simulink model "Three0mniwheel"  (R2020a)
settings: Solver=VariableStepAuto  StartTime=0.0  StopTime=inf  RelTol=1e-3
values from neighbouring files (symbols this model uses):
  sampleTime = 0.05    [PR_TR_parameters.m]
libraries: mobileRoboticsLib x4
settings Model: Creator=ADMIN  LastModifiedBy=RAJENDRA PHUTANE

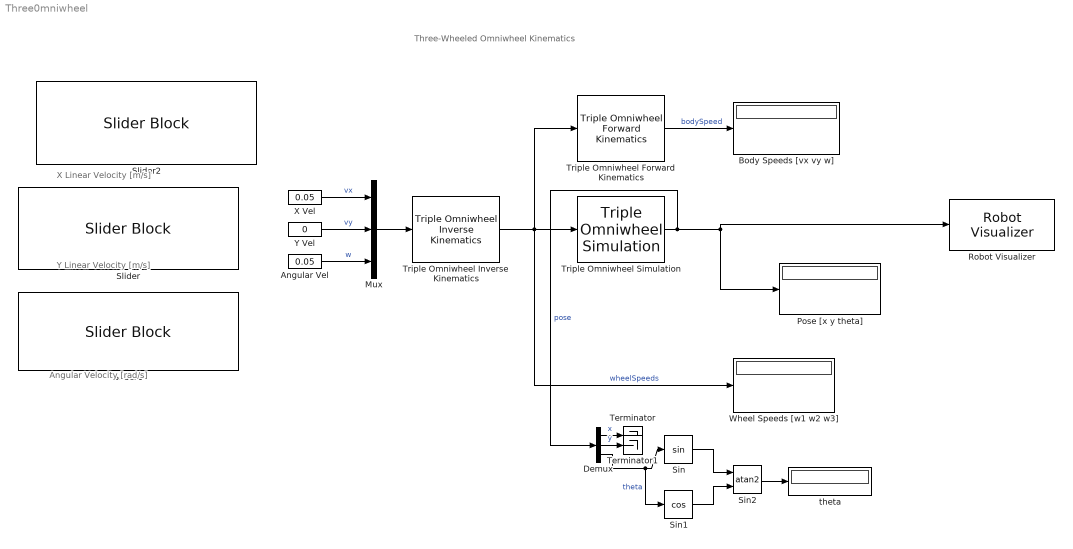
== system Three0mniwheel ==
  note: Angular Velocity [rad/s]
  note: Y Linear Velocity [m/s]
  note: Three-Wheeled Omniwheel Kinematics
  note: X Linear Velocity [m/s]
  Angular Vel : Constant  Value=0.05
  Body Speeds [vx vy w] : Display
  Demux : Demux  Outputs=3
  Mux : Mux  Inputs=3
  Pose [x y theta] : Display
  Robot Visualizer : mobileRoboticsLib/Environments/Robot Visualizer  Priority=99  robotRadius=TR.RobotRadius  mapName=arena_map_small  showTrajectory=on  hasWaypoints=off  hasLidar=off  sensorOffset=[ 0 0 ]  scanAngles=scanAngles  hasObjDetector=off  objDetectorOffset=[ 0, 0 ]  objDetectorAngle=0  objDetectorFOV=pi/4  objDetectorMaxRange=5  objectColors=[ 1, 0, 0; 0, 1, 0; 0, 0, 1 ]  objectMarkers=s
      settings: SourceProductName=Ground Vehicles Library
  Sin : Trigonometry  OutputSignalType=real
  Sin1 : Trigonometry  Operator=cos  OutputSignalType=real
  Sin2 : Trigonometry  Operator=atan2  OutputSignalType=real
  Slider : SliderBlock  ScaleMin=-1  ScaleMax=1  TickInterval=0.25
  Slider1 : SliderBlock  ScaleMin=-1.5  ScaleMax=1.5
  Slider2 : SliderBlock  ScaleMin=-1  ScaleMax=1  TickInterval=0.25
  Terminator : Terminator
  Terminator1 : Terminator
  Triple Omniwheel Forward Kinematics : mobileRoboticsLib/Kinematic Models/Triple Omniwheel/Triple Omniwheel Forward Kinematics  wheelRadius=TR.wheelRadius  robotRadius=TR.robotPosition  wheelAngles=TR.wheelAngles
      settings: SourceProductName=Mobile Robotics Simulation Library
  "Triple Omniwheel Inverse Kinematics " : mobileRoboticsLib/Kinematic Models/Triple Omniwheel/Triple Omniwheel Inverse Kinematics   wheelRadius=TR.wheelRadius  robotRadius=TR.robotPosition  wheelAngles=TR.wheelAngles
      settings: SourceProductName=Mobile Robotics Simulation Library
  Triple Omniwheel Simulation : mobileRoboticsLib/Kinematic Models/Triple Omniwheel/Triple Omniwheel Simulation  wheelRadius=TR.wheelRadius  robotRadius=TR.robotPosition  wheelAngles=TR.wheelAngles  initX=4  initY=4  initAngle=0  Ts=sampleTime
      settings: SourceProductName=Mobile Robotics Simulation Library
  Wheel Speeds [w1 w2 w3] : Display
  X Vel : Constant  Value=0.05
  Y Vel : Constant  Value=0
  theta : Display
  wires:
  Mux/1 -> "Triple Omniwheel Inverse Kinematics "/1
  Triple Omniwheel Simulation/1 -> Demux/1, Pose [x y theta]/1, Robot Visualizer/1  "pose"
  Y Vel/1 -> Mux/2  "vy"
  X Vel/1 -> Mux/1  "vx"
  Triple Omniwheel Forward Kinematics/1 -> Body Speeds [vx vy w]/1  "bodySpeed"
  "Triple Omniwheel Inverse Kinematics "/1 -> Triple Omniwheel Forward Kinematics/1, Triple Omniwheel Simulation/1, Wheel Speeds [w1 w2 w3]/1  "wheelSpeeds"
  Angular Vel/1 -> Mux/3  "w"
  Demux/1 -> Terminator/1  "x"
  Demux/2 -> Terminator1/1  "y"
  Demux/3 -> Sin1/1, Sin/1  "theta"
  Sin/1 -> Sin2/1
  Sin1/1 -> Sin2/2
  Sin2/1 -> theta/1
